simulink library "lib_etc"  (Simulink 4.1.1)
values from neighbouring files (symbols this model uses):
  logFlag = 1    [advSACompMaskInit.m]    (also in advSACompMaskInitR13.m)
undefined symbols (not defined in the file or in its folder): generalName, output_signal, time_signal_per_period
libraries: lib_fuel_converter x1
settings Model: LastModifiedBy=mokeefe
settings Model: ModifiedComment=|
  | mokeefe -- Tue Jan 21 11:27:07 2003 -- Version 1.47
  | added breakLinkCopyFcn as the copy script called by enhancedToWorkspace
settings Model: ModifiedHistory=|
  | mokeefe -- Tue Jan 21 11:27:07 2003 -- Version 1.47
  | added breakLinkCopyFcn as the copy script called by enhancedToWorkspace
  | 
  | mokeefe -- Tue Jan 21 11:27:07 2003 -- Version 1.47
  | added breakLinkCopyFcn as the copy script called by enhancedToWorkspace
  | 
  | mokeefe -- Tue Jan 21 11:23:26 2003 -- Version 1.46
  | added enhancedToWsMaker.m as the CopyFcn parameter for the enhancedToWorkspace block.
  | 
  | mokeefe -- Tue Jan 21 09:46:28 2003 -- Version 1.45
  | 
  | 
  | mokeefe -- Tue Jan 21 09:45:53 2003 -- Version 1.44
  | broke the enhancedToWorkspace inactive link to my test library (we want it to be resident in lib_etc.)
  | 
  | mokeefe -- Tue Jan 21 09:45:15 2003 -- Version 1.43
  | 
  | 
  | mokeefe -- Tue Jan 21 09:44:04 2003 -- Version 1.42
  | changed the enhancedToWorkspace block to work better--more rhobust
  | 
  | mokeefe -- Fri Jan 17 15:08:20 2003 -- Version 1.41
  | 
  | 
  | mokeefe -- Fri Jan 17 15:00:38 2003 -- Version 1.40
  | 
  | 
  | mokeefe -- Fri Jan 17 14:58:39 2003 -- Version 1.39
  | 
  | 
  | mokeefe -- Fri Jan 17 14:58:05 2003 -- Version 1.38
  | 
  | 
  | mokeefe -- Fri Jan 17 14:52:33 2003 -- Version 1.37
  | 
  | 
  | mokeefe -- Fri Jan 17 14:50:46 2003 -- Version 1.36
  | 
  | 
  | mokeefe -- Fri Jan 17 13:23:09 2003 -- Version 1.35
  | 
  | 
  | mokeefe -- Fri Jan 17 09:28:50 2003 -- Version 1.34
  | 
  | 
  | mokeefe -- Fri Jan 17 08:47:15 2003 -- Version 1.33
  | added enhancedToWorkspace block which allows you to log to the workspace and evaluate the variable name to use (while this is not as functional as the smartToWorkspace blocks, it is a simulink-only implimentation and is thus fast)
  | 
  | mokeefe -- Thu Dec 12 14:06:55 2002 -- Version 1.32
  | 
  | 
  | mokeefe -- Thu Dec 12 14:04:43 2002 -- Version 1.31
  | 
  | 
  | mokeefe -- Thu Dec 12 13:59:07 2002 -- Version 1.30
  | updated sfunSmartToWorkspace
  | This function now will only take one specific name and will place variables on the workspace as matrices (instead of just arrays)
  | 
  | mokeefe -- Thu Dec 12 13:24:20 2002 -- Version 1.29
  | 
  | 
  | mokeefe -- Thu Dec 12 13:20:31 2002 -- Version 1.28
  | 
  | 
  | mokeefe -- Thu Dec 12 13:19:14 2002 -- Version 1.27
  | 
  | 
  | mokeefe -- Thu Dec 12 11:45:14 2002 -- Version 1.26
  | 
  | 
  | mokeefe -- Thu Dec 12 11:39:22 2002 -- Version 1.25
  | 
  | 
  | mokeefe -- Thu Dec 12 11:12:09 2002 -- Version 1.24
  | 
  | 
  | mokeefe -- Thu Dec 12 11:11:12 2002 -- Version 1.23
  | 
  | 
  | mokeefe -- Thu Dec 12 10:56:47 2002 -- Version 1.22
  | finished sfunSmartToWorkspace
  | 
  | mokeefe -- Thu Dec 12 10:53:34 2002 -- Version 1.21
  | updated sfunSmartToWorkspace
  | 
  | mokeefe -- Thu Dec 12 10:44:52 2002 -- Version 1.20
  | Added an s-function version of smartToWorkspace to be used with subsystems
  | 
  | mokeefe -- Tue Apr 23 08:53:51 2002 -- Version 1.19
  | added filters against divide by zero or divide by zero or negative.
  | 
  | mokeefe -- Thu Apr 18 08:31:43 2002 -- Version 1.18
  | saving the model:
  | o "without the model browser open"
  | o with only top-level screen visible
  | o with "fit to view" enabled
  | o with "status bar" off and "toolbar" off
  | o with "prompt to update model history with each save" on

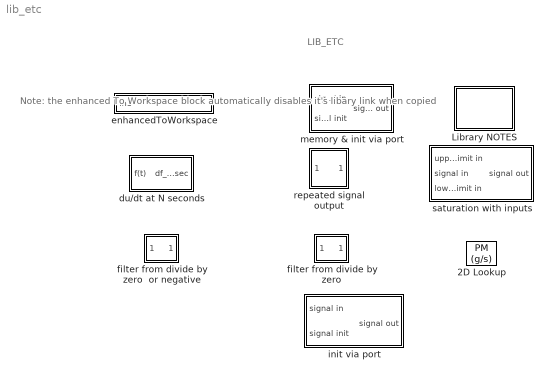
== system lib_etc ==
  note: LIB_ETC
  note: Note: the enhanced
      | To Workspace block
      | automatically disables
      | it's libary link when
      | copied
  2D Lookup : lib_fuel_converter/configurable subsystems/fuel use and EO emis Neural Network Model/HOT engine maps /PM (g//s)  MaskParam1=fc_map_spd*fc_spd_scale  MaskParam2=fc_map_trq*fc_trq_scale  MaskParam3=fc_pm_map*fc_spd_scale*fc_trq_scale
  Library NOTES : Subsystem
      settings: RTWFcnNameOpts=Auto  RTWFileNameOpts=Auto
      mask Display: disp('Library\nNOTES')
  du/dt at N seconds : Subsystem  mask{delay=5}
      mask prompts: delay "Delay (seconds)"
      settings: RTWFcnNameOpts=Auto  RTWFileNameOpts=Auto
  enhancedToWorkspace : Subsystem  TreatAsAtomicUnit=on  mask(enhancedToWorkspace){generalName=generalName, specificName=varName, logFlag=logFlag}
      mask prompts: generalName "General Name [char-evaluated]"; specificName "Specific Name [char-literal]"; logFlag "Enable flag (1=on,0=off)"
      mask help: A wrapper for the Simulink "To Workspace" block that allows you to evaluate the name of the variable to log to workspace. This is useful to avoid the double logging errors that occur when you pull in two library models that attempt to log to the same variable.
      mask init:
      | enhancedToWsMaker
      settings: CopyFcn=breakLinkCopyFcn  ParentCloseFcn=breakLinkParCloseFcn  RTWFcnNameOpts=Auto  RTWFileNameOpts=Auto
      mask Help:
      | <h2>Enhanced To Workspace Block</h2>
      | <h3>Parameters</h3>
      | <UL>
      | <li><b>General Name:</b> This is the more general name of the variable. Variables are saved to the workspace as <i>generalName_specificName</i>. Note that this is an evaluated variable. If you would like to type in the value directly, it must be surrounded with single quotes. Otherwise you can input the name of a variable containing a char string.</li>
      | <li><b>Specific Name:</b> This is the specific name of the variable. Note that this is input as a char literal (i.e., you don't need quotes).</li>
      | <li><b>Enable Flag:</b> This flag should have the value of 0 or 1. If 0, the variable will not be logged to the workspace. If 1, the variable will be logged. This is done so that variable logging can be turned off to improve speed.</li>
      | </ul>
      | <h3>Overview</h3>
      | <p>The enhanced to workspace block was put together to allow one to dynamically resolve variable names at run time in simulink. This is most powerful when used in conjunction with a masked subsystem to allow multiple instances of that masked subsytem to be used in the same model. The strategy is to set the generalName in the block mask which will allow the block to change the general name for all variable logging on the fly.
      | <h3>Helper Files</h3>
      | <p>Three m-files are required by the enhancedToWorkspace block. These files are located in the &lt; ADVISOR root &gt;/GUI directory :
      | <ul>
      | <li><i>enhancedToWsMaker.m</i> This file runs the mask initialization for the block</li>
      | <li><i>breakLinkCopyFcn.m</i> This file is used by the block callback when the simulink block is copied. It is necessary to break the link to the enhancedToWorkspace similar to the To Workspace block in order for it to be able to configure itself. (Try copying simulink's To Workspace block--it is impossible to make a link)</li>
      | <li><i>breakLinkParCloseFcn.m</i> This file is similar to the breakLinkCopyFcn and is used when a parent system is closed</li>
      | </ul>
      | <hr>
      | 
      | <p>Created 2003-Jan-21, Michael Patrick O'Keefe, NREL</p>
      | 
      | <!--
      | <VARDEF>
      | <H3>var_name</H3>
      | <UL>
      | <LI><B>data type</B> data type here</LI>
      | <LI><B>units</B> units here</LI>
      | <LI><B>vehicle type</B> vehicle type here</LI>
      | <LI><B>description</B> description here</LI>
      | </UL>
      | </VARDEF>
      | -->
      mask Display: disp([generalName,'_',specificName])
  filter from divide by zero : Subsystem
      settings: RTWFcnNameOpts=Auto  RTWFileNameOpts=Auto
  "filter from divide by zero  or negative " : Subsystem
      settings: RTWFcnNameOpts=Auto  RTWFileNameOpts=Auto
  init via port : Subsystem
      settings: RTWFcnNameOpts=Auto  RTWFileNameOpts=Auto
  memory & init via port : Subsystem
      settings: RTWFcnNameOpts=Auto  RTWFileNameOpts=Auto
  repeated signal output : Subsystem  mask(Repeating table){t=time_signal_per_period, y=output_signal}
      mask prompts: t "Input values:"; y "Output values:"
      mask help:
      | Repeating table.
      | Enter values of input and output for first cycle.
      mask init:
      | period = max(@1);
      settings: RTWFcnNameOpts=Auto  RTWFileNameOpts=Auto
      mask Help: Repeats signal given in table over time period given by the time signal. Input values should be monotonically increasing.
  saturation with inputs : Subsystem
      settings: RTWFcnNameOpts=Auto  RTWFileNameOpts=Auto

== system lib_etc/Library NOTES ==
  note: This library contains useful blocks that are used in other ADVISOR libraries but
      | do not necessarily have any direct relation to vehicles, the vehicle powertrain, or
      | powertrain components.

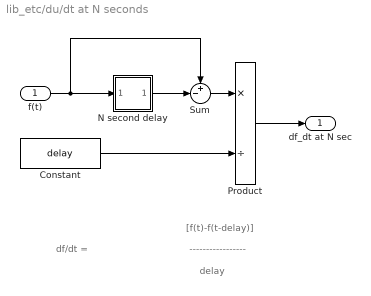
== system lib_etc/du/dt at N seconds ==
  note: [f(t)-f(t-delay)]
  note: -----------------
  note: delay
  note: df/dt =
  f(t) : Inport  Port=1  LatchInput=off
  Constant : Constant  Value=delay
  N second delay : Subsystem
      settings: RTWFcnNameOpts=Auto  RTWFileNameOpts=Auto
  Product : Product  Inputs=*/  Multiplication=Element-wise(.*)  SaturateOnIntegerOverflow=on
  Sum : Sum  Inputs=+-|  SaturateOnIntegerOverflow=on
  df_dt at N sec : Outport  Port=1
  wires:
  f(t)/1 -> Sum/1, N second delay/1(In1)
  Sum/1 -> Product/1
  Constant/1 -> Product/2
  Product/1 -> df_dt at N sec/1
  N second delay/1(Out1) -> Sum/2

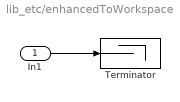
== system lib_etc/enhancedToWorkspace ==
  In1 : Inport  Port=1  LatchInput=off
  Terminator : Terminator
  wires:
  In1/1 -> Terminator/1

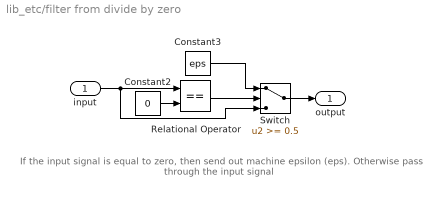
== system lib_etc/filter from divide by zero ==
  note: If the input signal is equal to zero,
      | then send out machine epsilon (eps). Otherwise
      | pass through the input signal
  input : Inport  Port=1  LatchInput=off
  Constant2 : Constant  Value=0
  Constant3 : Constant  Value=eps
  Relational Operator : RelationalOperator  Operator===
  Switch : Switch  Threshold=0.5
  output : Outport  Port=1
  wires:
  input/1 -> Switch/3, Relational Operator/1
  Constant2/1 -> Relational Operator/2
  Relational Operator/1 -> Switch/2
  Constant3/1 -> Switch/1
  Switch/1 -> output/1

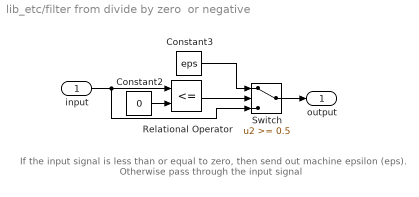
== system lib_etc/filter from divide by zero  or negative  ==
  note: If the input signal is less than or equal to zero,
      | then send out machine epsilon (eps). Otherwise
      | pass through the input signal
  input : Inport  Port=1  LatchInput=off
  Constant2 : Constant  Value=0
  Constant3 : Constant  Value=eps
  Relational Operator : RelationalOperator  Operator=<=
  Switch : Switch  Threshold=0.5
  output : Outport  Port=1
  wires:
  input/1 -> Switch/3, Relational Operator/1
  Constant2/1 -> Relational Operator/2
  Relational Operator/1 -> Switch/2
  Constant3/1 -> Switch/1
  Switch/1 -> output/1

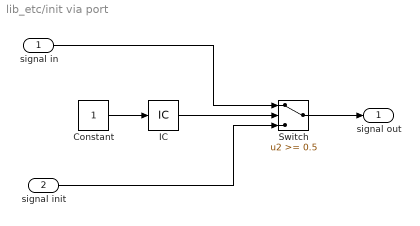
== system lib_etc/init via port ==
  signal in : Inport  Port=1  LatchInput=off
  signal init : Inport  Port=2  LatchInput=off
  Constant : Constant  Value=1
  IC : InitialCondition  Value=0
  Switch : Switch  Threshold=0.5
  signal out : Outport  Port=1
  wires:
  signal init/1 -> Switch/3
  Switch/1 -> signal out/1
  IC/1 -> Switch/2
  Constant/1 -> IC/1
  signal in/1 -> Switch/1

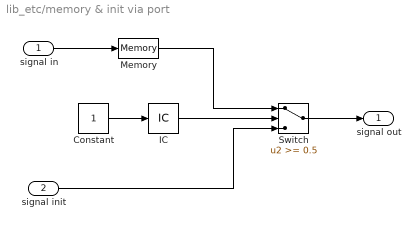
== system lib_etc/memory & init via port ==
  signal in : Inport  Port=1  LatchInput=off
  signal init : Inport  Port=2  LatchInput=off
  Constant : Constant  Value=1
  IC : InitialCondition  Value=0
  Memory : Memory  X0=0  InheritSampleTime=off
      settings: RTWStateStorageClass=Auto
  Switch : Switch  Threshold=0.5
  signal out : Outport  Port=1
  wires:
  signal in/1 -> Memory/1
  Constant/1 -> IC/1
  Memory/1 -> Switch/1
  IC/1 -> Switch/2
  Switch/1 -> signal out/1
  signal init/1 -> Switch/3

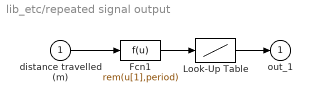
== system lib_etc/repeated signal output ==
  distance travelled (m) : Inport  Port=1  LatchInput=off
  Fcn1 : Fcn  Expr=rem(u[1],period)
  Look-Up Table : Lookup  InputValues=t  OutputValues=y
  out_1 : Outport  Port=1  InitialOutput=0
  wires:
  distance travelled (m)/1 -> Fcn1/1
  Fcn1/1 -> Look-Up Table/1
  Look-Up Table/1 -> out_1/1

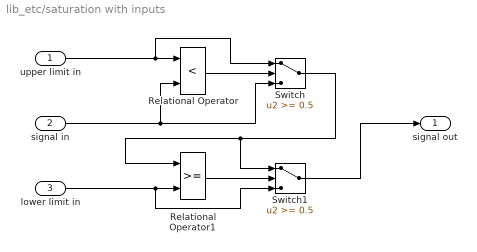
== system lib_etc/saturation with inputs ==
  upper limit in : Inport  Port=1  LatchInput=off
  signal in : Inport  Port=2  LatchInput=off
  lower limit in : Inport  Port=3  LatchInput=off
  Relational Operator : RelationalOperator  Operator=<
  Relational Operator1 : RelationalOperator  Operator=>=
  Switch : Switch  Threshold=0.5
  Switch1 : Switch  Threshold=0.5
  signal out : Outport  Port=1
  wires:
  upper limit in/1 -> Relational Operator/1, Switch/1
  lower limit in/1 -> Relational Operator1/2, Switch1/3
  Relational Operator/1 -> Switch/2
  Relational Operator1/1 -> Switch1/2
  Switch1/1 -> signal out/1
  signal in/1 -> Relational Operator/2, Switch/3
  Switch/1 -> Relational Operator1/1, Switch1/1

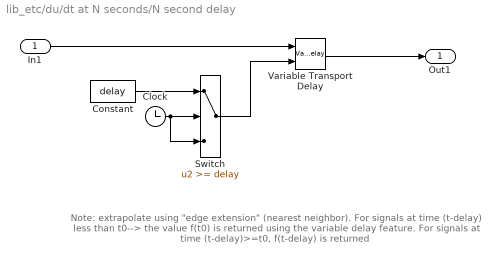
== system lib_etc/du/dt at N seconds/N second delay ==
  note: Note: extrapolate using "edge extension" (nearest neighbor).
      | For signals at time (t-delay) less than t0--> the value f(t0) is returned using the
      | variable delay feature. For signals at time (t-delay)>=t0, f(t-delay) is returned
  In1 : Inport  Port=1  LatchInput=off
  Clock : Clock
      settings: DisplayTime=off
  Constant : Constant  Value=delay
  Switch : Switch  Threshold=delay
  Variable Transport Delay : VariableTransportDelay  MaximumDelay=delay  InitialInput=0  MaximumPoints=1024  PadeOrder=0
  Out1 : Outport  Port=1
  wires:
  Clock/1 -> Switch/2, Switch/3
  In1/1 -> Variable Transport Delay/1
  Variable Transport Delay/1 -> Out1/1
  Switch/1 -> Variable Transport Delay/2
  Constant/1 -> Switch/1
